simulink library "aerosimlib"  (Simulink 5.0)
values from neighbouring files (symbols this model uses):
  stdatm = [0 100 200 300 400 500 600 700 800 900 1000 1100 ... (4305 elements, 861x5)]    [stdatm.mat]
undefined symbols (not defined in the file or in its folder): AlphaBnd, b, BetaBnd, CDda, CDde, CDdf, CDdr, CDM, CDmin, CGempty, CGgross, CL0, CLa, CLalphadot, Clbeta, Clda, CLde, CLdf, Cldr, CLM, CLmind, Clp, CLq, Clr, Cm0, Cma, Cmalphadot, Cmde, Cmdf, CmM, Cmq, Cnbeta, Cnda, Cndr, Cnp, Cnr, CP, CT, CYbeta, CYda, CYdr, CYp, CYr, Displacement, dmy, Engine, EulerIni, FuelFlow, FuelIni, J, Jempty, Jeng, Jgross, Jprop, MAC, MAP, MAPLim, MassIni, MaxPower, mempty ... (+25)
libraries: aerosimlib x350, simulink3 x41
(part 3 of 10)

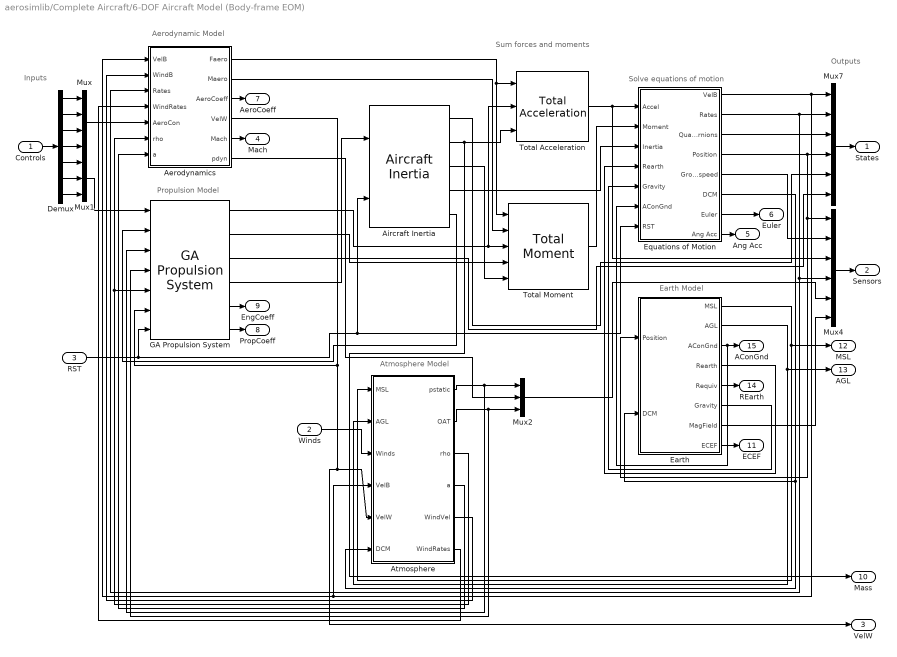
== system aerosimlib/Complete Aircraft/6-DOF Aircraft Model (Body-frame EOM) ==
  note: Propulsion Model
  note: Atmosphere Model
  note: Sum forces and moments
  note: Earth Model
  note: Aerodynamic Model
  note: Outputs
  note: Inputs
  note: Solve equations of motion
  Controls : Inport
  Winds : Inport  Port=2
  RST : Inport  Port=3
  Aerodynamics : Subsystem
  Aircraft Inertia : aerosimlib/Inertia/Aircraft Inertia  FuelIni=FuelIni  Mempty=mempty  Mgross=mgross  CGempty=CGempty  CGgross=CGgross  Jempty=Jempty  Jgross=Jgross
  Atmosphere : Subsystem
  Demux : Demux  Outputs=7
  Earth : Subsystem
  Equations of Motion : Subsystem
  GA Propulsion System : aerosimlib/Propulsion/GA Propulsion System  OmegaIni=OmegaIni  RPM=RPM  MAP=MAP  FuelFlow=FuelFlow  Power=Power  Jeng=Jeng  J=J  CT=CT  CP=CP  Rprop=Rprop  Jprop=Jprop  TSL=TSL
  Mux : Mux
  Mux1 : Mux  Inputs=3
  Mux2 : Mux  Inputs=3
  Mux4 : Mux  Inputs=6
  Mux7 : Mux  Inputs=6
  Total Acceleration : aerosimlib/Equations of Motion/Total Acceleration
  Total Moment : aerosimlib/Equations of Motion/Total Moment  raero=rAC  rprop=rHub
  States : Outport
  Sensors : Outport  Port=2
  VelW : Outport  Port=3
  Mach : Outport  Port=4
  Ang Acc : Outport  Port=5
  Euler : Outport  Port=6
  AeroCoeff : Outport  Port=7
  PropCoeff : Outport  Port=8
  EngCoeff : Outport  Port=9
  Mass : Outport  Port=10
  ECEF : Outport  Port=11
  MSL : Outport  Port=12
  AGL : Outport  Port=13
  REarth : Outport  Port=14
  AConGnd : Outport  Port=15
  wires:
  Earth/8(ECEF) -> ECEF/1
  Aerodynamics/3(AeroCoeff) -> AeroCoeff/1
  Aerodynamics/5(Mach) -> Mach/1
  Equations of Motion/3(Quaternions) -> Mux7/3
  Mux/1 -> Aerodynamics/5(AeroCon)
  Equations of Motion/4(Position) -> Mux7/4, Mux4/1, Earth/1(Position)
  Equations of Motion/2(Rates) -> Mux7/2, Mux4/4, Aerodynamics/3(Rates)
  Equations of Motion/1(VelB) -> Mux7/1, Atmosphere/4(VelB), Aerodynamics/1(VelB)
  Mux1/1 -> GA Propulsion System/1
  Mux7/1 -> States/1
  Mux4/1 -> Sensors/1
  Controls/1 -> Demux/1
  Demux/1 -> Mux/1
  Demux/2 -> Mux/2
  Demux/3 -> Mux/3
  Demux/4 -> Mux/4
  Demux/5 -> Mux1/1
  Demux/6 -> Mux1/2
  Demux/7 -> Mux1/3
  GA Propulsion System/5 -> EngCoeff/1
  GA Propulsion System/6 -> PropCoeff/1
  Earth/5(Requiv) -> REarth/1
  Earth/3(AConGnd) -> AConGnd/1, Equations of Motion/6(AConGnd)
  Equations of Motion/5(Groundspeed) -> Mux4/2
  Total Acceleration/1 -> Equations of Motion/1(Accel), Mux4/3
  Earth/7(MagField) -> Mux4/6
  Earth/6(Gravity) -> Equations of Motion/5(Gravity)
  Earth/4(Rearth) -> Equations of Motion/4(Rearth)
  Aircraft Inertia/2 -> Total Acceleration/3, Mass/1
  Aircraft Inertia/4 -> Equations of Motion/3(Inertia)
  Total Moment/1 -> Equations of Motion/2(Moment)
  Aircraft Inertia/3 -> Total Moment/5
  Aerodynamics/1(Faero) -> Total Acceleration/1, Total Moment/1
  Aerodynamics/2(Maero) -> Total Moment/2
  GA Propulsion System/1 -> Total Acceleration/2, Total Moment/3
  GA Propulsion System/2 -> Total Moment/4
  Equations of Motion/6(DCM) -> Earth/2(DCM), Atmosphere/6(DCM)
  Atmosphere/1(pstatic) -> Mux2/1, GA Propulsion System/3
  Atmosphere/2(OAT) -> Mux2/3, GA Propulsion System/4
  Aerodynamics/6(pdyn) -> Mux2/2
  Mux2/1 -> Mux4/5
  Aircraft Inertia/1 -> Mux7/5
  GA Propulsion System/3 -> Mux7/6
  GA Propulsion System/4 -> Aircraft Inertia/1
  Aerodynamics/4(VelW) -> GA Propulsion System/6, Atmosphere/5(VelW), VelW/1
  Earth/1(MSL) -> Atmosphere/1(MSL), MSL/1
  Earth/2(AGL) -> Atmosphere/2(AGL), AGL/1
  Winds/1 -> Atmosphere/3(Winds)
  Atmosphere/5(WindVel) -> Aerodynamics/2(WindB)
  Atmosphere/3(rho) -> Aerodynamics/6(rho), GA Propulsion System/5
  Atmosphere/4(a) -> Aerodynamics/7(a)
  Aircraft Inertia/5 -> GA Propulsion System/2
  RST/1 -> GA Propulsion System/7, Equations of Motion/7(RST), Aircraft Inertia/2
  Atmosphere/6(WindRates) -> Aerodynamics/4(WindRates)
  Equations of Motion/8(Ang Acc) -> Ang Acc/1
  Equations of Motion/7(Euler) -> Euler/1

== system aerosimlib/Complete Aircraft/6-DOF Aircraft Model (Geodetic-frame EOM) ==
  note: Propulsion Model
  note: Atmosphere Model
  note: Sum forces and moments
  note: Earth Model
  note: Aerodynamic Model
  note: Outputs
  note: Inputs
  note: Solve equations of motion
  Controls : Inport
  Winds : Inport  Port=2
  RST : Inport  Port=3
  Aerodynamics : Subsystem
  Aircraft Inertia : aerosimlib/Inertia/Aircraft Inertia  FuelIni=FuelIni  Mempty=mempty  Mgross=mgross  CGempty=CGempty  CGgross=CGgross  Jempty=Jempty  Jgross=Jgross
  Atmosphere : Subsystem
  Demux : Demux  Outputs=7
  Earth : Subsystem
  Equations of Motion : Subsystem
  GA Propulsion System : aerosimlib/Propulsion/GA Propulsion System  OmegaIni=OmegaIni  RPM=RPM  MAP=MAP  FuelFlow=FuelFlow  Power=Power  Jeng=Jeng  J=J  CT=CT  CP=CP  Rprop=Rprop  Jprop=Jprop  TSL=TSL
  Mux : Mux
  Mux1 : Mux  Inputs=3
  Mux2 : Mux  Inputs=3
  Mux4 : Mux  Inputs=6
  Mux7 : Mux  Inputs=6
  Total Acceleration : aerosimlib/Equations of Motion/Total Acceleration
  Total Moment : aerosimlib/Equations of Motion/Total Moment  raero=rAC  rprop=rHub
  States : Outport
  Sensors : Outport  Port=2
  VelW : Outport  Port=3
  Mach : Outport  Port=4
  Ang Acc : Outport  Port=5
  Euler : Outport  Port=6
  AeroCoeff : Outport  Port=7
  PropCoeff : Outport  Port=8
  EngCoeff : Outport  Port=9
  Mass : Outport  Port=10
  ECEF : Outport  Port=11
  MSL : Outport  Port=12
  AGL : Outport  Port=13
  REarth : Outport  Port=14
  AConGnd : Outport  Port=15
  wires:
  Earth/8(ECEF) -> ECEF/1
  Aerodynamics/3(AeroCoeff) -> AeroCoeff/1
  Aerodynamics/5(Mach) -> Mach/1
  Mux/1 -> Aerodynamics/5(AeroCon)
  Equations of Motion/5(Pos) -> Mux4/1, Earth/1(Position), Mux7/1
  Equations of Motion/3(Rates) -> Mux4/4, Aerodynamics/3(Rates), Mux7/4
  Equations of Motion/1(VelB) -> Atmosphere/4(VelB), Aerodynamics/1(VelB)
  Mux1/1 -> GA Propulsion System/1
  Mux7/1 -> States/1
  Mux4/1 -> Sensors/1
  Controls/1 -> Demux/1
  Demux/1 -> Mux/1
  Demux/2 -> Mux/2
  Demux/3 -> Mux/3
  Demux/4 -> Mux/4
  Demux/5 -> Mux1/1
  Demux/6 -> Mux1/2
  Demux/7 -> Mux1/3
  GA Propulsion System/5 -> EngCoeff/1
  GA Propulsion System/6 -> PropCoeff/1
  Earth/5(Requiv) -> REarth/1
  Earth/3(AConGnd) -> AConGnd/1, Equations of Motion/6(AConGnd)
  Equations of Motion/6(Groundspeed) -> Mux4/2
  Total Acceleration/1 -> Equations of Motion/1(Accel), Mux4/3
  Earth/7(MagField) -> Mux4/6
  Earth/6(Gravity) -> Equations of Motion/5(Gravity)
  Earth/4(Rearth) -> Equations of Motion/4(Rearth)
  Aircraft Inertia/2 -> Total Acceleration/3, Mass/1
  Aircraft Inertia/4 -> Equations of Motion/3(Inertia)
  Total Moment/1 -> Equations of Motion/2(Moment)
  Aircraft Inertia/3 -> Total Moment/5
  Aerodynamics/1(Faero) -> Total Acceleration/1, Total Moment/1
  Aerodynamics/2(Maero) -> Total Moment/2
  GA Propulsion System/1 -> Total Acceleration/2, Total Moment/3
  GA Propulsion System/2 -> Total Moment/4
  Equations of Motion/7(DCM) -> Earth/2(DCM), Atmosphere/6(DCM)
  Atmosphere/1(pstatic) -> Mux2/1, GA Propulsion System/3
  Atmosphere/2(OAT) -> Mux2/3, GA Propulsion System/4
  Aerodynamics/6(pdyn) -> Mux2/2
  Mux2/1 -> Mux4/5
  Aircraft Inertia/1 -> Mux7/5
  GA Propulsion System/3 -> Mux7/6
  GA Propulsion System/4 -> Aircraft Inertia/1
  Aerodynamics/4(VelW) -> GA Propulsion System/6, Atmosphere/5(VelW), VelW/1
  Earth/1(MSL) -> Atmosphere/1(MSL), MSL/1
  Earth/2(AGL) -> Atmosphere/2(AGL), AGL/1
  Winds/1 -> Atmosphere/3(Winds)
  Atmosphere/5(WindVel) -> Aerodynamics/2(WindB)
  Atmosphere/3(rho) -> Aerodynamics/6(rho), GA Propulsion System/5
  Atmosphere/4(a) -> Aerodynamics/7(a)
  Aircraft Inertia/5 -> GA Propulsion System/2
  RST/1 -> GA Propulsion System/7, Equations of Motion/7(RST), Aircraft Inertia/2
  Atmosphere/6(WindRates) -> Aerodynamics/4(WindRates)
  Equations of Motion/9(Ang Acc) -> Ang Acc/1
  Equations of Motion/8(Euler) -> Euler/1
  Equations of Motion/2(VelNED) -> Mux7/2
  Equations of Motion/4(Quaternions) -> Mux7/3

== system aerosimlib/Complete Aircraft/6-DOF Aircraft Model (Geodetic-frame EOM) No magnetic field ==
  note: Solve equations of motion
  note: Inputs
  note: Outputs
  note: Aerodynamic Model
  note: Earth Model
  note: Sum forces and moments
  note: Atmosphere Model
  note: Propulsion Model
  Controls : Inport
  Winds : Inport  Port=2
  RST : Inport  Port=3
  Aerodynamics : Subsystem
  Aircraft Inertia : aerosimlib/Inertia/Aircraft Inertia  FuelIni=FuelIni  Mempty=mempty  Mgross=mgross  CGempty=CGempty  CGgross=CGgross  Jempty=Jempty  Jgross=Jgross
  Atmosphere : Subsystem
  Demux : Demux  Outputs=7
  Earth : Subsystem
  Equations of Motion : Subsystem
  GA Propulsion System : aerosimlib/Propulsion/GA Propulsion System  OmegaIni=OmegaIni  RPM=RPM  MAP=MAP  FuelFlow=FuelFlow  Power=Power  Jeng=Jeng  J=J  CT=CT  CP=CP  Rprop=Rprop  Jprop=Jprop  TSL=TSL
  Mux : Mux
  Mux1 : Mux  Inputs=3
  Mux2 : Mux  Inputs=3
  Mux4 : Mux  Inputs=5
  Mux7 : Mux  Inputs=6
  Total Acceleration : aerosimlib/Equations of Motion/Total Acceleration
  Total Moment : aerosimlib/Equations of Motion/Total Moment  raero=rAC  rprop=rHub
  States : Outport
  Sensors : Outport  Port=2
  VelW : Outport  Port=3
  Mach : Outport  Port=4
  Ang Acc : Outport  Port=5
  Euler : Outport  Port=6
  AeroCoeff : Outport  Port=7
  PropCoeff : Outport  Port=8
  EngCoeff : Outport  Port=9
  Mass : Outport  Port=10
  ECEF : Outport  Port=11
  MSL : Outport  Port=12
  AGL : Outport  Port=13
  REarth : Outport  Port=14
  AConGnd : Outport  Port=15
  wires:
  Equations of Motion/4(Quaternions) -> Mux7/3
  Equations of Motion/2(VelNED) -> Mux7/2
  Equations of Motion/8(Euler) -> Euler/1
  Equations of Motion/9(Ang Acc) -> Ang Acc/1
  Atmosphere/6(WindRates) -> Aerodynamics/4(WindRates)
  RST/1 -> Aircraft Inertia/2, Equations of Motion/7(RST), GA Propulsion System/7
  Aircraft Inertia/5 -> GA Propulsion System/2
  Atmosphere/4(a) -> Aerodynamics/7(a)
  Atmosphere/3(rho) -> GA Propulsion System/5, Aerodynamics/6(rho)
  Atmosphere/5(WindVel) -> Aerodynamics/2(WindB)
  Winds/1 -> Atmosphere/3(Winds)
  Earth/2(AGL) -> AGL/1, Atmosphere/2(AGL)
  Earth/1(MSL) -> MSL/1, Atmosphere/1(MSL)
  Aerodynamics/4(VelW) -> VelW/1, Atmosphere/5(VelW), GA Propulsion System/6
  GA Propulsion System/4 -> Aircraft Inertia/1
  GA Propulsion System/3 -> Mux7/6
  Aircraft Inertia/1 -> Mux7/5
  Mux2/1 -> Mux4/5
  Aerodynamics/6(pdyn) -> Mux2/2
  Atmosphere/2(OAT) -> GA Propulsion System/4, Mux2/3
  Atmosphere/1(pstatic) -> GA Propulsion System/3, Mux2/1
  Equations of Motion/7(DCM) -> Atmosphere/6(DCM)
  GA Propulsion System/2 -> Total Moment/4
  GA Propulsion System/1 -> Total Acceleration/2, Total Moment/3
  Aerodynamics/1(Faero) -> Total Acceleration/1, Total Moment/1
  Aircraft Inertia/3 -> Total Moment/5
  Total Moment/1 -> Equations of Motion/2(Moment)
  Aircraft Inertia/4 -> Equations of Motion/3(Inertia)
  Aircraft Inertia/2 -> Total Acceleration/3, Mass/1
  Earth/4(Rearth) -> Equations of Motion/4(Rearth)
  Earth/6(Gravity) -> Equations of Motion/5(Gravity)
  Total Acceleration/1 -> Mux4/3, Equations of Motion/1(Accel)
  Equations of Motion/6(Groundspeed) -> Mux4/2
  Earth/3(AConGnd) -> Equations of Motion/6(AConGnd), AConGnd/1
  Earth/5(Requiv) -> REarth/1
  GA Propulsion System/6 -> PropCoeff/1
  GA Propulsion System/5 -> EngCoeff/1
  Demux/7 -> Mux1/3
  Demux/6 -> Mux1/2
  Demux/5 -> Mux1/1
  Demux/4 -> Mux/4
  Demux/3 -> Mux/3
  Demux/2 -> Mux/2
  Demux/1 -> Mux/1
  Controls/1 -> Demux/1
  Mux4/1 -> Sensors/1
  Mux7/1 -> States/1
  Mux1/1 -> GA Propulsion System/1
  Equations of Motion/1(VelB) -> Aerodynamics/1(VelB), Atmosphere/4(VelB)
  Equations of Motion/3(Rates) -> Mux7/4, Mux4/4, Aerodynamics/3(Rates)
  Equations of Motion/5(Pos) -> Mux7/1, Earth/1(Position), Mux4/1
  Mux/1 -> Aerodynamics/5(AeroCon)
  Aerodynamics/5(Mach) -> Mach/1
  Aerodynamics/3(AeroCoeff) -> AeroCoeff/1
  Earth/7(ECEF) -> ECEF/1
  Aerodynamics/2(Maero) -> Total Moment/2

== system aerosimlib/Complete Aircraft/Glider Model ==
  note: Sum forces and moments
  note: Aerodynamic Model
  note: Outputs
  note: Inputs
  note: Solve equations of motion
  Controls : Inport
  Aerodynamics : aerosimlib/Complete Aircraft/6-DOF Aircraft Model (Body-frame EOM)/Aerodynamics  SimViewingDevice=off
      settings: Permissions=ReadWrite  RTWFcnNameOpts=Auto  RTWFileNameOpts=Auto
  Aircraft Inertia : aerosimlib/Inertia/Aircraft Inertia  FuelIni=0  Mempty=mempty  Mgross=mgross  CGempty=CGempty  CGgross=CGgross  Jempty=Jempty  Jgross=Jgross
  Constant{,5,7..8} (4 alike) : Constant  Value=0
  Constant3 : Constant  Value=zeros(3,1)
  Constant4 : Constant  Value=zeros(3,1)
  Demux1 : Demux  Outputs=3
  Equations of Motion : Subsystem
  Mux2 : Mux  Inputs=3
  Mux3 : Mux  Orientation=left  Inputs=2
  Mux4 : Mux  Inputs=5
  Mux7 : Mux
  Standard Atmosphere : aerosimlib/Atmosphere/Standard Atmosphere
  Terminator{1..6} (6 alike) : Terminator
  Total Acceleration : aerosimlib/Equations of Motion/Total Acceleration
  Total Moment : aerosimlib/Equations of Motion/Total Moment  raero=rAC  rprop=rHub
  WGS-84 : aerosimlib/Earth/WGS-84  Orientation=left
  States : Outport
  Sensors : Outport  Port=2
  VelW : Outport  Port=3
  Mach : Outport  Port=4
  Ang Acc : Outport  Port=5
  Euler : Outport  Port=6
  AeroCoeff : Outport  Port=7
  wires:
  Aerodynamics/3 -> AeroCoeff/1
  Aerodynamics/5 -> Mach/1
  Equations of Motion/3(Quaternions) -> Mux7/3
  Equations of Motion/4(Position) -> Mux7/4, Mux4/1, Demux1/1, WGS-84/1
  Equations of Motion/2(Rates) -> Mux7/2, Mux4/4, Aerodynamics/3
  Equations of Motion/1(VelB) -> Mux7/1, Aerodynamics/1
  Mux7/1 -> States/1
  Mux4/1 -> Sensors/1
  Controls/1 -> Aerodynamics/5
  Equations of Motion/5(Groundspeed) -> Mux4/2
  Total Acceleration/1 -> Equations of Motion/1(Accel), Mux4/3
  Aircraft Inertia/2 -> Total Acceleration/3
  Aircraft Inertia/4 -> Equations of Motion/3(Inertia)
  Total Moment/1 -> Equations of Motion/2(Moment)
  Aircraft Inertia/3 -> Total Moment/5
  Aerodynamics/1 -> Total Acceleration/1, Total Moment/1
  Aerodynamics/2 -> Total Moment/2
  Aerodynamics/6 -> Mux2/2
  Mux2/1 -> Mux4/5
  Aerodynamics/4 -> VelW/1
  Equations of Motion/7(Euler) -> Euler/1
  Equations of Motion/8(Ang Acc) -> Ang Acc/1
  Constant/1 -> Equations of Motion/6(AConGnd)
  Constant7/1 -> Equations of Motion/7(RST)
  Equations of Motion/6(DCM) -> Terminator2/1
  Demux1/1 -> Terminator1/1
  Demux1/2 -> Terminator3/1
  Demux1/3 -> Standard Atmosphere/1
  Standard Atmosphere/1 -> Mux2/1
  Standard Atmosphere/2 -> Mux2/3
  Standard Atmosphere/3 -> Aerodynamics/6
  Standard Atmosphere/4 -> Aerodynamics/7
  Constant3/1 -> Aerodynamics/2
  Constant4/1 -> Aerodynamics/4
  Constant8/1 -> Aircraft Inertia/2
  Constant5/1 -> Aircraft Inertia/1
  Aircraft Inertia/5 -> Terminator4/1
  Aircraft Inertia/1 -> Terminator5/1
  WGS-84/1 -> Mux3/1
  WGS-84/2 -> Mux3/2
  WGS-84/3 -> Terminator6/1
  Mux3/1 -> Equations of Motion/4(Rearth)
  WGS-84/4 -> Equations of Motion/5(Gravity)

== system aerosimlib/Complete Aircraft/Inertial Navigation System ==
  IMU : Inport  PortDimensions=[6 1]  SampleTime=tsamp
  RST : Inport  Port=2  PortDimensions=1  SampleTime=tsamp
  Attitude : aerosimlib/Equations of Motion/Body-Frame EOM/Kinematics (Quaternions)  QuaternionsIni=QuaternionsIni
  Body-Inertial DCM : aerosimlib/Transformations/Body-Inertial DCM From Quaternions  Orientation=left
  Constant : Constant  Value=0
  Demux : Demux  Outputs=2
  Mux : Mux  Inputs=3
  Position : aerosimlib/Equations of Motion/Geodetic-Frame EOM/Position  PositionIni=PositionIni
  Terminator : Terminator
  Velocity : aerosimlib/Equations of Motion/Geodetic-Frame EOM/Velocity  VelocitiesIni=VelocitiesIni
  WGS-84 : aerosimlib/Earth/WGS-84
  PVA : Outport
  wires:
  IMU/1 -> Demux/1
  WGS-84/3 -> Terminator/1
  Velocity/1 -> Position/1, Mux/2
  WGS-84/1 -> Position/2
  WGS-84/2 -> Position/3
  WGS-84/4 -> Velocity/5
  Demux/1 -> Velocity/3
  Demux/2 -> Attitude/1
  RST/1 -> Attitude/2, Position/5, Velocity/6
  Attitude/1 -> Mux/3, Body-Inertial DCM/1
  Position/1 -> Velocity/1, WGS-84/1, Mux/1
  Position/2 -> Velocity/2
  Constant/1 -> Position/4
  Mux/1 -> PVA/1
  Body-Inertial DCM/1 -> Velocity/4

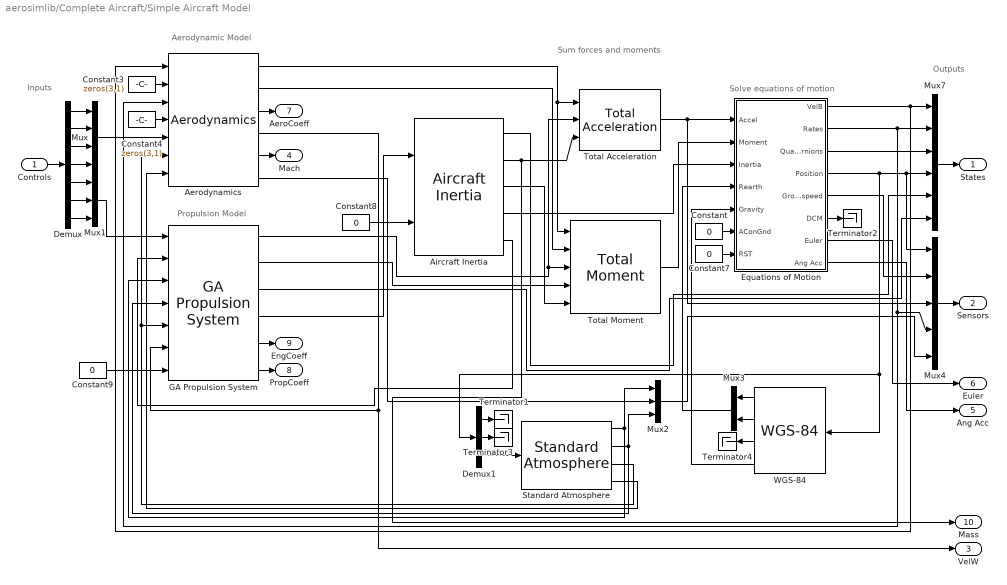
== system aerosimlib/Complete Aircraft/Simple Aircraft Model ==
  note: Propulsion Model
  note: Sum forces and moments
  note: Aerodynamic Model
  note: Outputs
  note: Inputs
  note: Solve equations of motion
  Controls : Inport
  Aerodynamics : aerosimlib/Complete Aircraft/6-DOF Aircraft Model (Body-frame EOM)/Aerodynamics  SimViewingDevice=off
      settings: Permissions=ReadWrite  RTWFcnNameOpts=Auto  RTWFileNameOpts=Auto
  Aircraft Inertia : aerosimlib/Inertia/Aircraft Inertia  FuelIni=FuelIni  Mempty=mempty  Mgross=mgross  CGempty=CGempty  CGgross=CGgross  Jempty=Jempty  Jgross=Jgross
  Constant{,7..9} (4 alike) : Constant  Value=0
  Constant3 : Constant  Value=zeros(3,1)
  Constant4 : Constant  Value=zeros(3,1)
  Demux : Demux  Outputs=7
  Demux1 : Demux  Outputs=3
  Equations of Motion : Subsystem
  GA Propulsion System : aerosimlib/Propulsion/GA Propulsion System  OmegaIni=OmegaIni  RPM=RPM  MAP=MAP  FuelFlow=FuelFlow  Power=Power  Jeng=Jeng  J=J  CT=CT  CP=CP  Rprop=Rprop  Jprop=Jprop  TSL=TSL
  Mux : Mux
  Mux1 : Mux  Inputs=3
  Mux2 : Mux  Inputs=3
  Mux3 : Mux  Orientation=left  Inputs=2
  Mux4 : Mux  Inputs=5
  Mux7 : Mux  Inputs=6
  Standard Atmosphere : aerosimlib/Atmosphere/Standard Atmosphere
  Terminator{1..4} (4 alike) : Terminator
  Total Acceleration : aerosimlib/Equations of Motion/Total Acceleration
  Total Moment : aerosimlib/Equations of Motion/Total Moment  raero=rAC  rprop=rHub
  WGS-84 : aerosimlib/Earth/WGS-84  Orientation=left
  States : Outport
  Sensors : Outport  Port=2
  VelW : Outport  Port=3
  Mach : Outport  Port=4
  Ang Acc : Outport  Port=5
  Euler : Outport  Port=6
  AeroCoeff : Outport  Port=7
  PropCoeff : Outport  Port=8
  EngCoeff : Outport  Port=9
  Mass : Outport  Port=10
  wires:
  Aerodynamics/3 -> AeroCoeff/1
  Aerodynamics/5 -> Mach/1
  Equations of Motion/3(Quaternions) -> Mux7/3
  Mux/1 -> Aerodynamics/5
  Equations of Motion/4(Position) -> Mux7/4, Mux4/1, Demux1/1, WGS-84/1
  Equations of Motion/2(Rates) -> Mux7/2, Mux4/4, Aerodynamics/3
  Equations of Motion/1(VelB) -> Mux7/1, Aerodynamics/1
  Mux1/1 -> GA Propulsion System/1
  Mux7/1 -> States/1
  Mux4/1 -> Sensors/1
  Controls/1 -> Demux/1
  Demux/1 -> Mux/1
  Demux/2 -> Mux/2
  Demux/3 -> Mux/3
  Demux/4 -> Mux/4
  Demux/5 -> Mux1/1
  Demux/6 -> Mux1/2
  Demux/7 -> Mux1/3
  GA Propulsion System/5 -> EngCoeff/1
  GA Propulsion System/6 -> PropCoeff/1
  Equations of Motion/5(Groundspeed) -> Mux4/2
  Total Acceleration/1 -> Equations of Motion/1(Accel), Mux4/3
  Aircraft Inertia/2 -> Mass/1, Total Acceleration/3
  Aircraft Inertia/4 -> Equations of Motion/3(Inertia)
  Total Moment/1 -> Equations of Motion/2(Moment)
  Aircraft Inertia/3 -> Total Moment/5
  Aerodynamics/1 -> Total Acceleration/1, Total Moment/1
  GA Propulsion System/1 -> Total Acceleration/2, Total Moment/3
  GA Propulsion System/2 -> Total Moment/4
  Aerodynamics/6 -> Mux2/2
  Mux2/1 -> Mux4/5
  Aircraft Inertia/1 -> Mux7/5
  GA Propulsion System/3 -> Mux7/6
  GA Propulsion System/4 -> Aircraft Inertia/1
  Aerodynamics/4 -> GA Propulsion System/6, VelW/1
  Aircraft Inertia/5 -> GA Propulsion System/2
  Equations of Motion/7(Euler) -> Euler/1
  Equations of Motion/8(Ang Acc) -> Ang Acc/1
  Constant/1 -> Equations of Motion/6(AConGnd)
  Constant7/1 -> Equations of Motion/7(RST)
  Equations of Motion/6(DCM) -> Terminator2/1
  Demux1/1 -> Terminator1/1
  Demux1/2 -> Terminator3/1
  Demux1/3 -> Standard Atmosphere/1
  Standard Atmosphere/1 -> Mux2/1, GA Propulsion System/3
  Standard Atmosphere/2 -> Mux2/3, GA Propulsion System/4
  Standard Atmosphere/3 -> Aerodynamics/6, GA Propulsion System/5
  Standard Atmosphere/4 -> Aerodynamics/7
  Constant3/1 -> Aerodynamics/2
  Constant4/1 -> Aerodynamics/4
  Constant8/1 -> Aircraft Inertia/2
  Constant9/1 -> GA Propulsion System/7
  Aerodynamics/2 -> Total Moment/2
  WGS-84/1 -> Mux3/1
  WGS-84/2 -> Mux3/2
  Mux3/1 -> Equations of Motion/4(Rearth)
  WGS-84/4 -> Equations of Motion/5(Gravity)
  WGS-84/3 -> Terminator4/1

== system aerosimlib/Earth/EGM-96 ==
  note: Sources
  note: Compute Mean-Sea Level Altitude
  Position : Inport
  Demux2 : Demux  Outputs=3
  Longitude Bound 0-2pi : Subsystem
      mask Type: Longitude bound
      mask Description: Bounds the longitude to [0, 2pi]. When 0 bound is exceeded the longitude wraps back to 2pi; when the 2pi bound is exceeded the longitude wraps back to 0.
  Look-Up Table (2-D) : Lookup2D  RowIndex=Lat  ColumnIndex=Lon  OutputValues=Alterr'  SaturateOnIntegerOverflow=on  InputSameDT=on
  Sum : Sum  Inputs=+++  SaturateOnIntegerOverflow=on  InputSameDT=on
  WGS-84 correction : Constant  Value=-0.53
  rad 2 deg : Subsystem
      mask Type: Radians to degrees
      mask Description: Convert radians to degrees.
      mask Display: disp('RAD DEG');
  rad 2 deg1 : Subsystem
      mask Type: Radians to degrees
      mask Description: Convert radians to degrees.
      mask Display: disp('RAD DEG');
  MSLAlt : Outport
  wires:
  Longitude Bound 0-2pi/1(Out) -> rad 2 deg1/1(In)
  Position/1 -> Demux2/1
  Demux2/3 -> Sum/1
  Demux2/1 -> rad 2 deg/1(In)
  Demux2/2 -> Longitude Bound 0-2pi/1(In)
  rad 2 deg/1(Out) -> Look-Up Table (2-D)/1
  rad 2 deg1/1(Out) -> Look-Up Table (2-D)/2
  Look-Up Table (2-D)/1 -> Sum/2
  WGS-84 correction/1 -> Sum/3
  Sum/1 -> MSLAlt/1

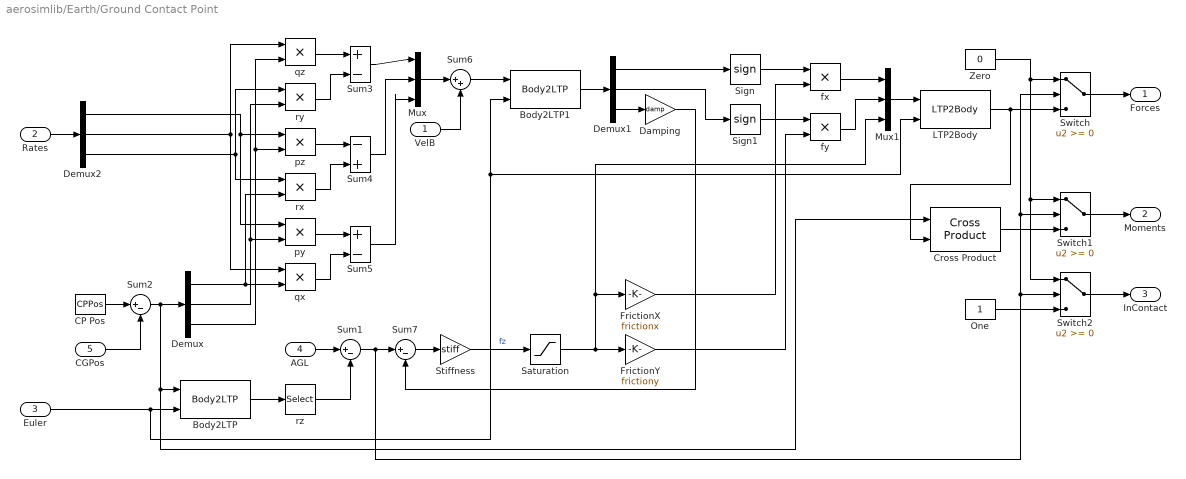
== system aerosimlib/Earth/Ground Contact Point ==
  VelB : Inport
  Rates : Inport  Port=2
  Euler : Inport  Port=3
  AGL : Inport  Port=4
  CGPos : Inport  Port=5
  Body2LTP : aerosimlib/Transformations/Body2LTP
  Body2LTP1 : aerosimlib/Transformations/Body2LTP
  CP Pos : Constant  Value=CPPos
  Cross Product : aerosimlib/Math/Cross Product
  Damping : Gain  Gain=damp  SaturateOnIntegerOverflow=on
  Demux : Demux  Outputs=3
  Demux1 : Demux  Outputs=3
  Demux2 : Demux  Outputs=3
  FrictionX : Gain  Gain=frictionx  SaturateOnIntegerOverflow=on
  FrictionY : Gain  Gain=frictiony  SaturateOnIntegerOverflow=on
  LTP2Body : aerosimlib/Transformations/LTP2Body
  Mux : Mux  Inputs=3
  Mux1 : Mux  Inputs=3
  One : Constant
  Saturation : Saturate  UpperLimit=0  LowerLimit=-Nmax
  Sign : Signum
  Sign1 : Signum
  Stiffness : Gain  Gain=stiff  SaturateOnIntegerOverflow=on
  Sum1 : Sum  Inputs=|+-  SaturateOnIntegerOverflow=on
  Sum2 : Sum  Inputs=|+-  SaturateOnIntegerOverflow=on
  Sum3 : Sum  Inputs=+-  SaturateOnIntegerOverflow=on
  Sum4 : Sum  Inputs=-+  SaturateOnIntegerOverflow=on
  Sum5 : Sum  Inputs=+-  SaturateOnIntegerOverflow=on
  Sum6 : Sum  Inputs=|++  SaturateOnIntegerOverflow=on
  Sum7 : Sum  Inputs=|+-  SaturateOnIntegerOverflow=on
  Switch : Switch  SaturateOnIntegerOverflow=on
  Switch1 : Switch  SaturateOnIntegerOverflow=on
  Switch2 : Switch  SaturateOnIntegerOverflow=on
  Zero : Constant  Value=0
  fx : Product  SaturateOnIntegerOverflow=on
  fy : Product  SaturateOnIntegerOverflow=on
  py : Product  SaturateOnIntegerOverflow=on
  pz : Product  SaturateOnIntegerOverflow=on
  qx : Product  SaturateOnIntegerOverflow=on
  qz : Product  SaturateOnIntegerOverflow=on
  rx : Product  SaturateOnIntegerOverflow=on
  ry : Product  SaturateOnIntegerOverflow=on
  rz : Selector  Elements=3  InputPortWidth=3
  Forces : Outport
  Moments : Outport  Port=2
  InContact : Outport  Port=3
  wires:
  Zero/1 -> Switch/1, Switch1/1, Switch2/1
  Switch1/1 -> Moments/1
  Switch/1 -> Forces/1
  Cross Product/1 -> Switch1/3
  LTP2Body/1 -> Switch/3, Cross Product/2
  Mux1/1 -> LTP2Body/1
  fy/1 -> Mux1/2
  fx/1 -> Mux1/1
  FrictionY/1 -> fy/2
  Sign1/1 -> fy/1
  FrictionX/1 -> fx/2
  Sign/1 -> fx/1
  Stiffness/1 -> Saturation/1  "fz"
  Demux1/2 -> Sign1/1
  Demux1/1 -> Sign/1
  Sum7/1 -> Stiffness/1
  Damping/1 -> Sum7/2
  Sum1/1 -> Sum7/1, Switch1/2, Switch/2, Switch2/2
  Demux1/3 -> Damping/1
  Body2LTP1/1 -> Demux1/1
  Sum6/1 -> Body2LTP1/1
  rz/1 -> Sum1/2
  Body2LTP/1 -> rz/1
  Euler/1 -> Body2LTP1/2, LTP2Body/2, Body2LTP/2
  VelB/1 -> Sum6/2
  Mux/1 -> Sum6/1
  Sum5/1 -> Mux/3
  Sum4/1 -> Mux/2
  Sum3/1 -> Mux/1
  qx/1 -> Sum5/2
  py/1 -> Sum5/1
  rx/1 -> Sum4/2
  pz/1 -> Sum4/1
  ry/1 -> Sum3/2
  qz/1 -> Sum3/1
  Demux2/1 -> py/1, pz/1
  Demux2/3 -> rx/1, ry/1
  Demux2/2 -> qx/1, qz/1
  CGPos/1 -> Sum2/2
  CP Pos/1 -> Sum2/1
  Sum2/1 -> Cross Product/1, Body2LTP/1, Demux/1
  Rates/1 -> Demux2/1
  AGL/1 -> Sum1/1
  Demux/3 -> pz/2, qz/2
  Demux/2 -> py/2, ry/2
  Demux/1 -> qx/2, rx/2
  Switch2/1 -> InContact/1
  One/1 -> Switch2/3
  Saturation/1 -> Mux1/3, FrictionX/1, FrictionY/1

== system aerosimlib/Earth/Ground Detection ==
  MSLAlt : Inport
  GndAlt : Inport  Port=2
  False : Constant  Value=0
  Sum : Sum  Inputs=|+-  SaturateOnIntegerOverflow=on  InputSameDT=on
  Switch : Switch  SaturateOnIntegerOverflow=on  InputSameDT=on
  True : Constant
  AConGnd : Outport
  AGLAlt : Outport  Port=2
  wires:
  MSLAlt/1 -> Sum/1
  GndAlt/1 -> Sum/2
  Sum/1 -> Switch/2, AGLAlt/1
  False/1 -> Switch/1
  True/1 -> Switch/3
  Switch/1 -> AConGnd/1

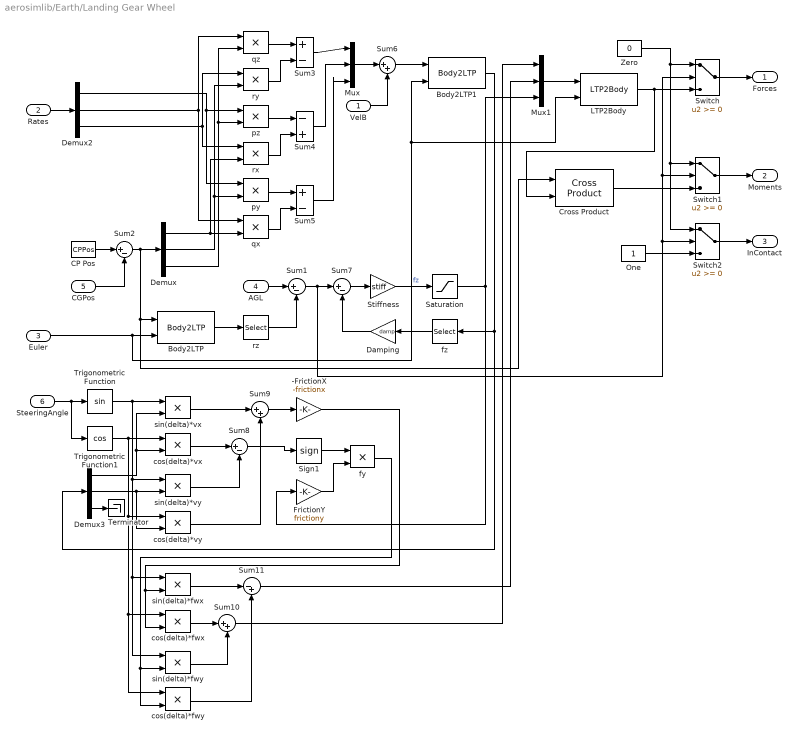
== system aerosimlib/Earth/Landing Gear Wheel ==
  VelB : Inport
  Rates : Inport  Port=2
  Euler : Inport  Port=3
  AGL : Inport  Port=4
  CGPos : Inport  Port=5
  SteeringAngle : Inport  Port=6
  -FrictionX : Gain  Gain=-frictionx  SaturateOnIntegerOverflow=on
  Body2LTP : aerosimlib/Transformations/Body2LTP
  Body2LTP1 : aerosimlib/Transformations/Body2LTP
  CP Pos : Constant  Value=CPPos
  Cross Product : aerosimlib/Math/Cross Product
  Damping : Gain  Orientation=left  Gain=damp  SaturateOnIntegerOverflow=on
  Demux : Demux  Outputs=3
  Demux2 : Demux  Outputs=3
  Demux3 : Demux  Outputs=3
  FrictionY : Gain  Gain=frictiony  SaturateOnIntegerOverflow=on
  LTP2Body : aerosimlib/Transformations/LTP2Body
  Mux : Mux  Inputs=3
  Mux1 : Mux  Inputs=3
  One : Constant
  Saturation : Saturate  UpperLimit=0  LowerLimit=-Nmax
  Sign1 : Signum
  Stiffness : Gain  Gain=stiff  SaturateOnIntegerOverflow=on
  Sum{1..2,7..8} (4 alike) : Sum  Inputs=|+-  SaturateOnIntegerOverflow=on
  Sum10 : Sum  Inputs=|++  SaturateOnIntegerOverflow=on
  Sum11 : Sum  Inputs=|-+  SaturateOnIntegerOverflow=on
  Sum3 : Sum  Inputs=+-  SaturateOnIntegerOverflow=on
  Sum4 : Sum  Inputs=-+  SaturateOnIntegerOverflow=on
  Sum5 : Sum  Inputs=+-  SaturateOnIntegerOverflow=on
  Sum6 : Sum  Inputs=|++  SaturateOnIntegerOverflow=on
  Sum9 : Sum  Inputs=|++  SaturateOnIntegerOverflow=on
  Switch : Switch  SaturateOnIntegerOverflow=on
  Switch1 : Switch  SaturateOnIntegerOverflow=on
  Switch2 : Switch  SaturateOnIntegerOverflow=on
  Terminator : Terminator
  Trigonometric Function : Trigonometry
  Trigonometric Function1 : Trigonometry  Operator=cos
  Zero : Constant  Value=0
  cos(delta)*fwx : Product  SaturateOnIntegerOverflow=on
  cos(delta)*fwy : Product  SaturateOnIntegerOverflow=on
  cos(delta)*vx : Product  SaturateOnIntegerOverflow=on
  cos(delta)*vy : Product  SaturateOnIntegerOverflow=on
  fy : Product  SaturateOnIntegerOverflow=on
  fz : Selector  Orientation=left  Elements=3  InputPortWidth=3
  py : Product  SaturateOnIntegerOverflow=on
  pz : Product  SaturateOnIntegerOverflow=on
  qx : Product  SaturateOnIntegerOverflow=on
  qz : Product  SaturateOnIntegerOverflow=on
  rx : Product  SaturateOnIntegerOverflow=on
  ry : Product  SaturateOnIntegerOverflow=on
  rz : Selector  Elements=3  InputPortWidth=3
  sin(delta)*fwx : Product  SaturateOnIntegerOverflow=on
  sin(delta)*fwy : Product  SaturateOnIntegerOverflow=on
  sin(delta)*vx : Product  SaturateOnIntegerOverflow=on
  sin(delta)*vy : Product  SaturateOnIntegerOverflow=on
  Forces : Outport
  Moments : Outport  Port=2
  InContact : Outport  Port=3
  wires:
  Demux/1 -> rx/2, qx/2
  Demux/2 -> ry/2, py/2
  Demux/3 -> qz/2, pz/2
  AGL/1 -> Sum1/1
  Rates/1 -> Demux2/1
  Sum2/1 -> Demux/1, Body2LTP/1, Cross Product/1
  CP Pos/1 -> Sum2/1
  CGPos/1 -> Sum2/2
  Demux2/2 -> qz/1, qx/1
  Demux2/3 -> ry/1, rx/1
  Demux2/1 -> pz/1, py/1
  qz/1 -> Sum3/1
  ry/1 -> Sum3/2
  pz/1 -> Sum4/1
  rx/1 -> Sum4/2
  py/1 -> Sum5/1
  qx/1 -> Sum5/2
  Sum3/1 -> Mux/1
  Sum4/1 -> Mux/2
  Sum5/1 -> Mux/3
  Mux/1 -> Sum6/1
  VelB/1 -> Sum6/2
  Euler/1 -> Body2LTP/2, LTP2Body/2, Body2LTP1/2
  Body2LTP/1 -> rz/1
  rz/1 -> Sum1/2
  Sum6/1 -> Body2LTP1/1
  Body2LTP1/1 -> Demux3/1, fz/1
  Sum1/1 -> Sum7/1, Switch/2, Switch1/2, Switch2/2
  Sum7/1 -> Stiffness/1
  Stiffness/1 -> Saturation/1  "fz"
  Mux1/1 -> LTP2Body/1
  LTP2Body/1 -> Cross Product/2, Switch/3
  Cross Product/1 -> Switch1/3
  Switch/1 -> Forces/1
  Switch1/1 -> Moments/1
  Zero/1 -> Switch/1, Switch1/1, Switch2/1
  SteeringAngle/1 -> Trigonometric Function/1, Trigonometric Function1/1
  Trigonometric Function/1 -> sin(delta)*vx/1, sin(delta)*vy/1, sin(delta)*fwx/1, sin(delta)*fwy/1
  Trigonometric Function1/1 -> cos(delta)*vx/1, cos(delta)*vy/1, cos(delta)*fwx/1, cos(delta)*fwy/1
  Demux3/1 -> sin(delta)*vx/2, cos(delta)*vx/2
  Demux3/2 -> sin(delta)*vy/2, cos(delta)*vy/2
  Demux3/3 -> Terminator/1
  cos(delta)*vx/1 -> Sum8/1
  sin(delta)*vy/1 -> Sum8/2
  sin(delta)*vx/1 -> Sum9/1
  cos(delta)*vy/1 -> Sum9/2
  Sum9/1 -> -FrictionX/1
  Sum8/1 -> Sign1/1
  Sign1/1 -> fy/1
  FrictionY/1 -> fy/2
  -FrictionX/1 -> cos(delta)*fwx/2, sin(delta)*fwx/2
  fy/1 -> cos(delta)*fwy/2, sin(delta)*fwy/2
  cos(delta)*fwx/1 -> Sum10/1
  sin(delta)*fwy/1 -> Sum10/2
  sin(delta)*fwx/1 -> Sum11/1
  cos(delta)*fwy/1 -> Sum11/2
  Sum10/1 -> Mux1/1
  Sum11/1 -> Mux1/2
  Damping/1 -> Sum7/2
  fz/1 -> Damping/1
  Switch2/1 -> InContact/1
  One/1 -> Switch2/3
  Saturation/1 -> FrictionY/1, Mux1/3

== system aerosimlib/Earth/WGS-84 ==
  note: Sources
  note: Compute radii and surface gravity
  note: Correct gravity for altitude
  note: Outputs
  Position : Inport
  1/2 : Constant  Value=1/2
  3/2 : Constant  Value=3/2
  Demux2 : Demux  Outputs=3
  Equatorial Radius : Constant  Value=6378137
  First Eccentricity : Constant  Value=0.0818191908426
  Gravity at Equator : Constant  Value=9.7803267714
  Gravity formula const : Constant  Value=0.00193185138639
  Math Function : Math  Operator=pow
  Math Function1 : Math  Operator=pow
  Mux : Mux  Inputs=3
  One : Constant
  Product : Product  SaturateOnIntegerOverflow=on  InputSameDT=on
  Product1 : Product  Inputs=**/  SaturateOnIntegerOverflow=on  InputSameDT=on
  Product2 : Product  Inputs=*/  SaturateOnIntegerOverflow=on  InputSameDT=on
  Product3 : Product  SaturateOnIntegerOverflow=on  InputSameDT=on
  Product4 : Product  Inputs=**/  SaturateOnIntegerOverflow=on  InputSameDT=on
  Product5 : Product  SaturateOnIntegerOverflow=on  InputSameDT=on
  Sum : Sum  Inputs=|+-  SaturateOnIntegerOverflow=on  InputSameDT=on
  Sum1 : Sum  Inputs=|+-  SaturateOnIntegerOverflow=on  InputSameDT=on
  Sum2 : Sum  Inputs=|++  SaturateOnIntegerOverflow=on  InputSameDT=on
  Terminator : Terminator
  eps^2 : Math  Operator=square
  g(phi,h) : Fcn  Expr=u[1]-(3.0877e-6 - 0.0044e-6*u[2])*u[3]+0.072e-12*u[3]*u[3]
  sin(phi) : Trigonometry
  sin(phi)^2 : Math  Operator=square
  sqrt : Math  Operator=sqrt
  Rmeridian : Outport
  Rnormal : Outport  Port=2
  Re : Outport  Port=3
  Gravity : Outport  Port=4
  wires:
  sqrt/1 -> Re/1
  Product5/1 -> sqrt/1
  First Eccentricity/1 -> eps^2/1
  eps^2/1 -> Sum/2, Product/1
  sin(phi)/1 -> sin(phi)^2/1
  sin(phi)^2/1 -> Product/2, Product3/2, Mux/2
  One/1 -> Sum1/1, Sum2/1, Sum/1
  Product/1 -> Sum1/2
  Sum1/1 -> Math Function/1, Math Function1/1
  3/2/1 -> Math Function/2
  1/2/1 -> Math Function1/2
  Equatorial Radius/1 -> Product1/1, Product2/1
  Sum/1 -> Product1/2
  Math Function/1 -> Product1/3
  Math Function1/1 -> Product2/2, Product4/3
  Product1/1 -> Rmeridian/1, Product5/1
  Product2/1 -> Rnormal/1, Product5/2
  Gravity formula const/1 -> Product3/1
  Product3/1 -> Sum2/2
  Gravity at Equator/1 -> Product4/1
  Sum2/1 -> Product4/2
  Product4/1 -> Mux/1
  Position/1 -> Demux2/1
  Demux2/1 -> sin(phi)/1
  Demux2/2 -> Terminator/1
  Mux/1 -> g(phi,h)/1
  g(phi,h)/1 -> Gravity/1
  Demux2/3 -> Mux/3

== system aerosimlib/Earth/WMM-2000 ==
  Position : Inport  PortDimensions=[3 1]  DataType=double
  DCM : Inport  Port=2  PortDimensions=[3 3]  DataType=double
  Date : Constant  Value=simdate
  DayToYear : Gain  Gain=1/365  SaturateOnIntegerOverflow=on
  Demux : Demux  Outputs=3
  Demux1 : Demux  Outputs=3
  MonthToYear : Gain  Gain=1/12  SaturateOnIntegerOverflow=on
  Mux : Mux  Inputs=3
  Product : Product  Multiplication=Matrix(*)  SaturateOnIntegerOverflow=on  InputSameDT=on
  S-Function : S-Function  FunctionName=sfunwmm  Parameters=wmmfile
  Sum : Sum  Inputs=+++  SaturateOnIntegerOverflow=on  InputSameDT=on
  MagField : Outport
  wires:
  S-Function/1 -> Product/2
  DCM/1 -> Product/1
  Date/1 -> Demux/1
  Demux/1 -> DayToYear/1
  DayToYear/1 -> Sum/1
  Demux/2 -> MonthToYear/1
  Demux/3 -> Sum/3
  MonthToYear/1 -> Sum/2
  Position/1 -> S-Function/1
  Sum/1 -> S-Function/2
  Product/1 -> Demux1/1
  Demux1/1 -> Mux/1
  Demux1/2 -> Mux/2
  Demux1/3 -> Mux/3
  Mux/1 -> MagField/1

== system aerosimlib/Equations of Motion/Body-Frame EOM ==
  Forces : Subsystem  mask(Force equations){VelocitiesIni=VelocitiesIni}
      mask prompts: VelocitiesIni "Initial velocities:"
      mask help: 6-DOF rigid body force equations.
      mask Help:
      | The block implements the 6-DOF rigid-body force equations.
      | <P><B>Inputs:</B>
      | <LI>Rates = the 3x1 vector of body angular rates</LI>
      | <LI>Accel = the 3x1 vector of linear body accelerations</LI>
      | <LI>Gravity = the gravitational acceleration at current location.
      | <LI>DCM = the 3x3 rotation matrix from navigation to body frame.
      | <LI>RST = the integrator reset flag (rising edge)</LI>
      | </P>
      | <P><B>Output:</B>
      | <LI>Velocities = the 3x1 vector of aircraft velocities in body axes</LI>
      | </P>
      | <P><B>Parameters:</B>
      | <LI>Initial velocities = the 3x1 vector of initial aircraft velocities</LI>
      | </P>
  Kinematics (Euler) : Subsystem  mask(Kinematic Equations){EulerIni=EulerIni}
      mask prompts: EulerIni "Initial Euler angles:"
      mask help: 6-DOF rigid body kinematic equations, using Euler angles.
      mask Help:
      | The block implements the 6-DOF rigid-body kinematic equations, using Euler angles.
      | <P><B>Inputs:</B>
      | <LI>Rates = the 3x1 vector of body angular rates</LI>
      | <LI>RST = the integrator reset flag (rising edge)</LI>
      | </P>
      | <P><B>Output:</B>
      | <LI>Euler = the 3x1 vector of Euler angles</LI>
      | </P>
      | <P><B>Parameters:</B>
      | <LI>Initial Euler angles = the 3x1 vector of initial body attitude</LI>
      | </P>
  Kinematics (Quaternions) : Subsystem  mask(Kinematic Equations){QuaternionsIni=QuaternionsIni}
      mask prompts: QuaternionsIni "Initial quaternions:"
      mask help: 6-DOF rigid body kinematic equations, using Euler-Rodrigues quaternions.
      mask Help:
      | The block implements the 6-DOF rigid-body kinematic equations, using Euler-Rodrigues quaternions.
      | <P><B>Inputs:</B>
      | <LI>Rates = the 3x1 vector of body angular rates</LI>
      | <LI>RST = the integrator reset flag (rising edge)</LI>
      | </P>
      | <P><B>Output:</B>
      | <LI>Quaternions = the 4x1 vector of body quaternions</LI>
      | </P>
      | <P><B>Parameters:</B>
      | <LI>Initial quaternions = the 4x1 vector of initial body quaternions</LI>
      | </P>
  Moments : Subsystem  mask(Moment equations){RatesIni=RatesIni}
      mask prompts: RatesIni "Initial angular rates:"
      mask help: 6-DOF rigid body moment equations.
      mask Help:
      | The block implements the 6-DOF rigid-body moment equations.
      | <P><B>Inputs:</B>
      | <LI>Inertia = the 10x1 vector of inertia coefficients</LI>
      | <LI>Moments = the 3x1 vector of airframe moments</LI>
      | <LI>RST = the integrator reset flag (rising edge)</LI>
      | </P>
      | <P><B>Output:</B>
      | <LI>Angular Rates = the 3x1 vector of body angular rates</LI>
      | <LI>Angular Acc = the 3x1 vector of body angular accelerations.
      | </P>
      | <P><B>Parameters:</B>
      | <LI>Initial rates = the 3x1 vector of initial angular rates</LI>
      | </P>
  Navigation : Subsystem  mask(Navigation equations){PositionIni=PositionIni}
      mask prompts: PositionIni "Initial position:"
      mask help: 6-DOF rigid body navigation equations.
      mask Help:
      | The block implements the inertial navigation equations.
      | <P><B>Inputs:</B>
      | <LI>Velocities = the 3x1 vector of aircraft velocities in body axes</LI>
      | <LI>DCM = the 3x3 frame transformation from navigation frame to body frame</LI>
      | <LI>Rmeridian = the Earth meridian radius, in m</LI>
      | <LI>Rnormal = the Earth normal radius, in m</LI>
      | <LI>AConGnd = the aircraft-on-ground flag</LI>
      | <LI>RST = the integrator reset flag (rising edge)</LI>
      | </P>
      | <P><B>Output:</B>
      | <LI>Position = the 3x1 vector of aircraft location [Latitude Longitude Altitude] in [rad rad m]</LI>
      | <LI>Gndspd = the 3x1 vector of aircraft velocities in navigation frame [North East Down] in m/s</LI>
      | </P>
      | <P><B>Parameters:</B>
      | <LI>Initial position = the 3x1 vector of initial aircraft position</LI>
      | </P>

== system aerosimlib/Equations of Motion/Geodetic-Frame EOM ==
  Angular Rate : Subsystem  mask(Angular rate equations){RatesIni=}
      mask prompts: RatesIni "Initial angular rates:"
      mask help: The angular rate equations in body frame which take the Earth rotation rate into account.
      mask Help:
      | The block implements the body angular rate equations by integrating the moments applied to the airframe and adding the Earth rotation rate components in body axes.
      | <P><B>Inputs:</B>
      | <LI>Inertia = the 10x1 vector of inertia coefficients</LI>
      | <LI>Moments = the 3x1 vector of airframe moments</LI>
      | <LI>Pos = the 3x1 vector of aircraft geodetic position [Lat Lon Alt]
      | <LI>dPosdt = the 3x1 vector of aircraft position derivatives
      | <LI>DCM = the 3x3 navigation-to-body frame transformation matrix
      | <LI>RST = the integrator reset flag (rising edge)</LI>
      | </P>
      | <P><B>Output:</B>
      | <LI>Angular Rate = the 3x1 vector of body angular rates</LI>
      | <LI>Angular Acc = the 3x1 vector of body angular accelerations.
      | </P>
      | <P><B>Parameters:</B>
      | <LI>Initial rates = the 3x1 vector of initial angular rates</LI>
      | </P>
  Attitude (Euler) : aerosimlib/Equations of Motion/Body-Frame EOM/Kinematics (Euler)  EulerIni=EulerIni
  Attitude (Quaternions) : aerosimlib/Equations of Motion/Body-Frame EOM/Kinematics (Quaternions)  QuaternionsIni=QuaternionsIni
  Position : Subsystem  mask(Position equations){PositionIni=PositionIni}
      mask prompts: PositionIni "Initial position:"
      mask help: Position equations in geodetic frame. Assumes WGS-84 Earth geoid model.
      mask Help:
      | The block implements the inertial position equations in geodetic frame (North-East-Down).
      | <P><B>Inputs:</B>
      | <LI>Vel NED = the 3x1 vector of aircraft velocities in geodetic frame</LI>
      | <LI>Rmeridian = the Earth meridian radius, in m</LI>
      | <LI>Rnormal = the Earth normal radius, in m</LI>
      | <LI>AConGnd = the aircraft-on-ground flag</LI>
      | <LI>RST = the integrator reset flag (rising edge)</LI>
      | </P>
      | <P><B>Output:</B>
      | <LI>Position = the 3x1 vector of aircraft location [Latitude Longitude Altitude] in [rad rad m]</LI>
      | <LI>dPosdt = the 3x1 vector of aircraft position derivatives in m/s</LI>
      | </P>
      | <P><B>Parameters:</B>
      | <LI>Initial position = the 3x1 vector of initial aircraft position</LI>
      | </P>
  Velocity : Subsystem  mask(Velocity Equations){VelocitiesIni=VelocitiesIni}
      mask prompts: VelocitiesIni "Initial velocities:"
      mask help: The velocity equations in geodetic frame.
      mask Help:
      | The block implements the velocity equations in geodetic frame (North-East-Down).
      | <P><B>Inputs:</B>
      | <LI>Pos = the 3x1 vector of aircraft position [Lat Lon Alt];
      | <LI>dPosdt = the 3x1 vector of aircraft position derivatives;
      | <LI>Accel = the 3x1 vector of linear body accelerations</LI>
      | <LI>DCM = the 3x3 rotation matrix from navigation to body frame.
      | <LI>Gravity = the gravitational acceleration at current location.
      | <LI>RST = the integrator reset flag (rising edge)</LI>
      | </P>
      | <P><B>Output:</B>
      | <LI>Velocity NED = the 3x1 vector of aircraft velocities in geodetic frame</LI>
      | </P>
      | <P><B>Parameters:</B>
      | <LI>Initial velocities = the 3x1 vector of initial aircraft velocities in geodetic frame</LI>
      | </P>

== system aerosimlib/Equations of Motion/Total Acceleration ==
  note: Sources
  Faero : Inport  PortDimensions=[3 1]
  Fprop : Inport  Port=2  PortDimensions=[3 1]
  Mass : Inport  Port=3  PortDimensions=1
  F/m : Product  Inputs=*/  SaturateOnIntegerOverflow=on  InputSameDT=on
  Sum1 : Sum  SaturateOnIntegerOverflow=on  InputSameDT=on
  Acc : Outport
  wires:
  F/m/1 -> Acc/1
  Mass/1 -> F/m/2
  Sum1/1 -> F/m/1
  Fprop/1 -> Sum1/2
  Faero/1 -> Sum1/1

== system aerosimlib/Equations of Motion/Total Moment ==
  note: Sources
  note: Moments at CG created by aero and propulsion forces
  note: Total moments at CG location
  Faero : Inport  PortDimensions=[3 1]
  Maero : Inport  Port=2  PortDimensions=[3 1]
  Fprop : Inport  Port=3  PortDimensions=[3 1]
  Mprop : Inport  Port=4  PortDimensions=[3 1]
  CGpos : Inport  Port=5  PortDimensions=[3 1]
  Aero Moment : Subsystem
  Propulsion Moment : Subsystem
  Sum : Sum  Inputs=|+-  SaturateOnIntegerOverflow=on  InputSameDT=on
  Sum1 : Sum  Inputs=++++  SaturateOnIntegerOverflow=on  InputSameDT=on
  Sum2 : Sum  Inputs=|+-  SaturateOnIntegerOverflow=on  InputSameDT=on
  r_aero : Constant  Value=raero
  r_prop : Constant  Value=rprop
  Mcg : Outport
  wires:
  Propulsion Moment/1(ProdVec) -> Sum1/4
  Maero/1 -> Sum1/1
  Fprop/1 -> Propulsion Moment/2(Vec2)
  Mprop/1 -> Sum1/3
  Aero Moment/1(ProdVec) -> Sum1/2
  Sum1/1 -> Mcg/1
  Faero/1 -> Aero Moment/2(Vec2)
  r_aero/1 -> Sum2/1
  r_prop/1 -> Sum/1
  CGpos/1 -> Sum2/2, Sum/2
  Sum/1 -> Propulsion Moment/1(Vec1)
  Sum2/1 -> Aero Moment/1(Vec1)

== system aerosimlib/FlightGear-Compatible/Aerodynamics ==
  Coefficient : Subsystem  BlockChoice=Value
      settings: TemplateBlock=self  MemberBlocks=Table,Value,Vector
  Table : Subsystem  mask(Aerodynamic coefficient: Table){Table=0}
      mask prompts: Table "Coefficient:"
      mask help: The block implements a 2-D look-up table aerodynamic coefficient.
      mask Help:
      | The block implements a 2-D look-up table aerodynamic coefficient.
      | <P><B>Inputs:</B>
      | <LI>RowParam = the row argument for the look-up table</LI>
      | <LI>ColParam = the column argument for the look-up table</LI>
      | </P>
      | <P><B>Outputs:</B>
      | <LI>Coeff = the aerodynamic coefficient</LI>
      | </P>
      | <P><B>Parameters:</B>
      | <LI>Coefficient = the Matlab structure for a table-coefficient.</LI>
      | </P>
  Value : Subsystem  mask(Aerodynamic coefficient: Value){Value=0}
      mask prompts: Value "Coefficient:"
      mask help: The block implements a scalar aerodynamic coefficient.
      mask Help:
      | The block implements a scalar aerodynamic coefficient.
      | <P><B>Inputs:</B>
      | <LI>RowParam = the input argument</LI>
      | </P>
      | <P><B>Outputs:</B>
      | <LI>Coeff = the aerodynamic coefficient</LI>
      | </P>
      | <P><B>Parameters:</B>
      | <LI>Coefficient = the Matlab value-coefficient structure</LI>
      | </P>
  Vector : Subsystem  mask(Aerodynamic coefficient: Vector){Vector=0}
      mask prompts: Vector "Coefficient:"
      mask help: The block implements a vector (1-D look-up-table) aerodynamic coefficient.
      mask Help:
      | The block implements a vector (1-D look-up-table) aerodynamic coefficient.
      | <P><B>Inputs:</B>
      | <LI>RowParam = the input argument</LI>
      | </P>
      | <P><B>Outputs:</B>
      | <LI>Coeff = the aerodynamic coefficient</LI>
      | </P>
      | <P><B>Parameters:</B>
      | <LI>Coefficient = the Matlab structure of a vector coefficient</LI>
      | </P>
